simulink model "PitchSys"  (R2017b)
settings: Solver=ode1  StartTime=0.00  StopTime=10.00  FixedStep=0.01  RelTol=1e-3  EnableMultiTasking=on
undefined symbols (not defined in the file): Jp, k_d, k_s, l2
settings Model: Creator=bjones  LastModifiedBy=Brian
settings DataIOCC: SaveFormat=Array  SignalLoggingSaveFormat=ModelDataLogs
settings OptimizationCC: BlockReduction=off  BooleanDataType=off  ExpressionDepthLimit=2147483647  LifeSpan=inf
settings DebuggingCC: SaveWithParameterizedLinksMsg=none  UnderspecifiedInitializationDetection=Classic  MergeDetectMultiDrivingBlocksExec=none  SignalResolutionControl=TryResolveAllWithWarning  MultiTaskDSMMsg=warning  MultiTaskCondExecSysMsg=none  FcnCallInpInsideContextMsg=warning  StateNameClashWarn=warning  SFUnexpectedBacktrackingDiag=warning  SFNoUnconditionalDefaultTransitionDiag=warning  SFExecutionAtInitializationDiag=none
settings HardwareCC: ProdBitPerPointer=32  ProdBitPerSizeT=32  ProdBitPerPtrDiffT=32  ProdLargestAtomicFloat=None  ProdIntDivRoundTo=Undefined  ProdEndianess=Unspecified  ProdWordSize=32  ProdHWDeviceType=32-bit Generic  TargetUnknown=on
settings ModelReferenceCC: PropagateSignalLabelsOutOfModel=off
settings CodeAppCC: StateflowObjectComments=on
settings GRTTargetCC: TargetLangStandard=C89/C90 (ANSI)  GeneratePreprocessorConditionals=Disable all  CombineOutputUpdateFcns=off  GRTInterface=on
settings ConfigComp: CovMetricSettings=dw  CovHtmlReporting=on  CovSaveCumulativeToWorkspaceVar=on  CovSaveSingleToWorkspaceVar=on  CovExternalEMLEnable=off  CovSFcnEnable=off

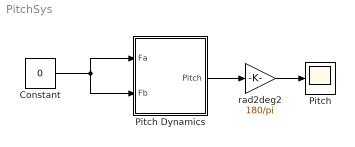
== system PitchSys ==
  Constant : Constant  Value=0
  Pitch : Scope
  Pitch Dynamics : Subsystem
  rad2deg2 : Gain  Gain=180/pi  SaturateOnIntegerOverflow=on  OutDataTypeStr=Inherit: Same as input  ParamDataTypeStr=Inherit: Same as input
  wires:
  Pitch Dynamics/1(Pitch) -> rad2deg2/1
  rad2deg2/1 -> Pitch/1
  Constant/1 -> Pitch Dynamics/1(Fa), Pitch Dynamics/2(Fb)

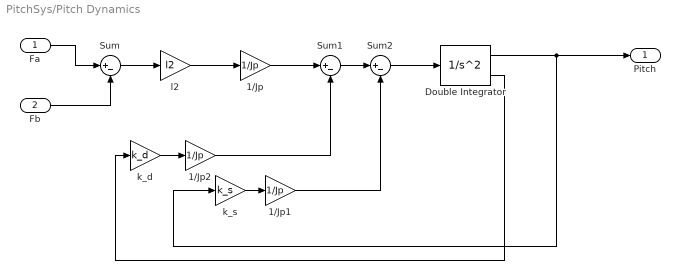
== system PitchSys/Pitch Dynamics ==
  Fa : Inport
  Fb : Inport  Port=2
  1/Jp : Gain  Gain=1/Jp
  1/Jp1 : Gain  Gain=1/Jp
  1/Jp2 : Gain  Gain=1/Jp
  Double Integrator : SecondOrderIntegrator  ICX=p_lim_u  LimitX=on  UpperLimitX=p_lim_u  LowerLimitX=p_lim_l
  Sum : Sum  Inputs=|+-
  Sum1 : Sum  Inputs=|+-
  Sum2 : Sum  Inputs=|+-
  k_d : Gain  Gain=k_d
  k_s : Gain  Gain=k_s
  l2 : Gain  Gain=l2
  Pitch : Outport
  wires:
  Double Integrator/1 -> k_s/1, Pitch/1
  Fa/1 -> Sum/1
  Fb/1 -> Sum/2
  Sum/1 -> l2/1
  k_d/1 -> 1/Jp2/1
  l2/1 -> 1/Jp/1
  k_s/1 -> 1/Jp1/1
  Sum1/1 -> Sum2/1
  Sum2/1 -> Double Integrator/1
  1/Jp1/1 -> Sum2/2
  1/Jp2/1 -> Sum1/2
  1/Jp/1 -> Sum1/1
  Double Integrator/2 -> k_d/1
